simulink model "TASK_42"  (R2018b)
settings: Solver=VariableStepAuto  StartTime=0.0  StopTime=10.0  MaxStep=1e-2  RelTol=1e-3
values from neighbouring files (symbols this model uses):
  A = [0 -168.333333333 0 111.111111111 1 -1.33333333333 0 2.77777777778 0 13.3333333333 0 -111.111111111 ... (16 elements, 4x4)]    [data.mat]
  B = [0  0; 0.0333333333333  0; 0  0; 0  0.277777777778]    [data.mat]
  C = [1 0 0 0 0 1 0 0 0 0 1 0 ... (16 elements, 4x4)]    [data.mat]
  D = [0  0; 0  0; 0  0; 0  0]    [data.mat]
libraries: slctrlblks x2
settings Model: Creator=Федор  LastModifiedBy=Федор

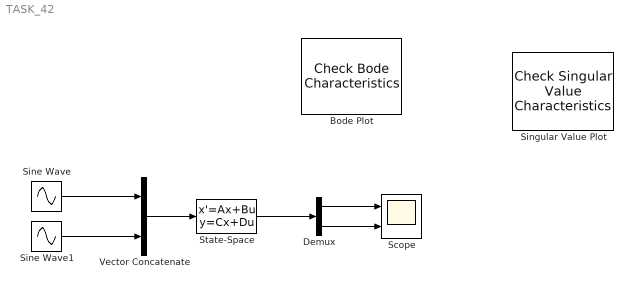
== system TASK_42 ==
  Bode Plot : slctrlblks/Model Verification/Check Bode  Characteristics  InstantiateOnLoad=on  SaveOperatingPoints=off  LinearizationIOs={'/Vector Concatenate', 1, 'in', 'off', '';'/State-Space', 1, 'out', 'off', ''}  LinearizeAt=SnapshotTimes  SnapshotTimes=[0]  TriggerType=rising  SampleTime=auto  RateConversionMethod=zoh  PreWarpFreq=10  UseExactDelayModel=off  UseFullBlockNameLabels=off  UseBusSignalLabels=off  enabled=on  stopWhenAssertionFail=off  export=off  ViewDlgPos=[1 41 1280 607.333333333333]  OpenViewOnLoad=off  LaunchViewOnOpen=on  FrequencyUnits=rad/s  MagnitudeUnits=dB  PhaseUnits=deg  TimeUnits=seconds  EnableUpperBound=off  UpperBoundFrequencies=[]  UpperBoundMagnitudes=[]  EnableLowerBound=off  LowerBoundFrequencies=[]  LowerBoundMagnitudes=[]
      settings: SourceProductName=Simulink Control Design
  Demux : Demux  Outputs=2
  Scope : Scope  NumInputPorts=2
  Sine Wave : Sin  Amplitude=5  Frequency=10  SampleTime=0
  Sine Wave1 : Sin  Amplitude=5  Frequency=10  SampleTime=0
  Singular Value Plot : slctrlblks/Model Verification/Check Singular Value Characteristics  InstantiateOnLoad=on  SaveOperatingPoints=off  LinearizationIOs={'/Vector Concatenate', 1, 'in', 'off', '';'/State-Space', 1, 'out', 'off', ''}  LinearizeAt=SnapshotTimes  SnapshotTimes=[0]  TriggerType=rising  SampleTime=auto  RateConversionMethod=zoh  PreWarpFreq=10  UseExactDelayModel=off  UseFullBlockNameLabels=off  UseBusSignalLabels=off  enabled=on  stopWhenAssertionFail=off  export=off  LaunchViewOnOpen=on  ViewDlgPos=[1 41 1280 607.333333333333]  OpenViewOnLoad=on  FrequencyUnits=rad/s  MagnitudeUnits=dB  PhaseUnits=deg  TimeUnits=seconds  EnableUpperBound=off  UpperBoundFrequencies=[]  UpperBoundMagnitudes=[]  EnableLowerBound=off  LowerBoundFrequencies=[]  LowerBoundMagnitudes=[]
      settings: SourceProductName=Simulink Control Design  SourceProductBaseCode=SD  SaveToWorkspace=off  SaveName=sys
  State-Space : StateSpace  A=A  B=B  C=C  D=D  InitialCondition=0
  Vector Concatenate : Concatenate
  wires:
  State-Space/1 -> Demux/1
  Vector Concatenate/1 -> State-Space/1
  Sine Wave/1 -> Vector Concatenate/1
  Sine Wave1/1 -> Vector Concatenate/2
  Demux/1 -> Scope/1
  Demux/2 -> Scope/2
